simulink model "SimplificationDemo_Before"  (Simulink 7.8)
settings: Solver=ode45  StartTime=0.0  StopTime=10.0  RelTol=1e-3
settings Model: Creator=760162  LastModifiedBy=monika

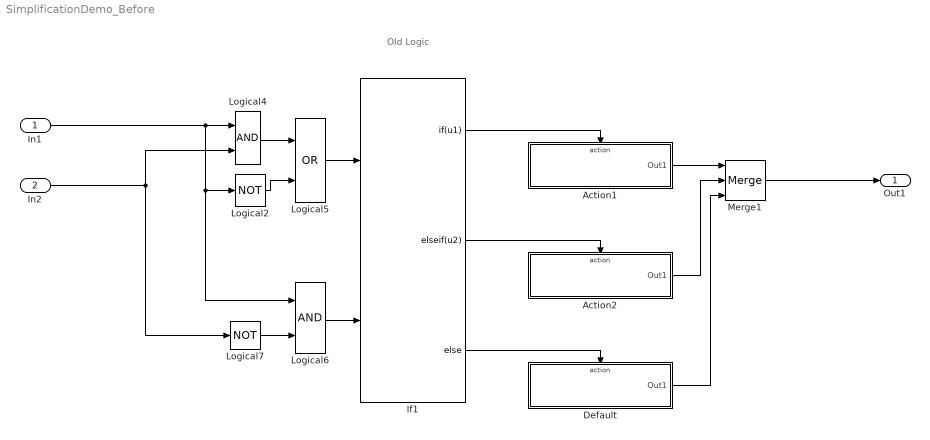
== system SimplificationDemo_Before ==
  note: Old Logic
  In1 : Inport
  In2 : Inport  Port=2
  Action1 : Subsystem  TreatAsAtomicUnit=on
      settings: CopyFcn=breaklink(gcb)  PropExecContextOutsideSubsystem=on
      mask Display:
      | text(.52,.01,char(get_param(gcb,'Tag') ), 'horizontalAlignment','center','verticalAlignment','bottom' )
      | disp(get_param(gcb,'Name'))
  Action2 : Subsystem  TreatAsAtomicUnit=on
      settings: CopyFcn=breaklink(gcb)  PropExecContextOutsideSubsystem=on
      mask Display:
      | text(.52,.01,char(get_param(gcb,'Tag') ), 'horizontalAlignment','center','verticalAlignment','bottom' )
      | disp(get_param(gcb,'Name'))
  Default : Subsystem  TreatAsAtomicUnit=on
      settings: CopyFcn=breaklink(gcb)  PropExecContextOutsideSubsystem=on
      mask Display:
      | text(.52,.01,char(get_param(gcb,'Tag') ), 'horizontalAlignment','center','verticalAlignment','bottom' )
      | disp(get_param(gcb,'Name'))
  If1 : If  NumInputs=2  IfExpression=u1  ElseIfExpressions=u2
      settings: CopyFcn=breaklink(gcb)
  Logical2 : Logic  Operator=NOT  OutDataTypeStr=boolean
  Logical4 : Logic  OutDataTypeStr=boolean
  Logical5 : Logic  Operator=OR  OutDataTypeStr=boolean
  Logical6 : Logic  OutDataTypeStr=boolean
  Logical7 : Logic  Operator=NOT  OutDataTypeStr=boolean
  Merge1 : Merge  Inputs=3
  Out1 : Outport
  wires:
  In1/1 -> Logical4/1, Logical6/1, Logical2/1
  Logical4/1 -> Logical5/1
  Logical5/1 -> If1/1
  Logical7/1 -> Logical6/2
  If1/1 -> Action1/Action
  If1/2 -> Action2/Action
  If1/3 -> Default/Action
  Logical6/1 -> If1/2
  Action1/1(Out1) -> Merge1/1
  Action2/1(Out1) -> Merge1/2
  Default/1(Out1) -> Merge1/3
  Merge1/1 -> Out1/1
  In2/1 -> Logical4/2, Logical7/1
  Logical2/1 -> Logical5/2

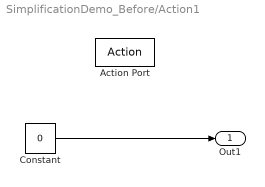
== system SimplificationDemo_Before/Action1 ==
  Action Port : ActionPort  ActionType=then
  Constant : Constant  Value=0
  Out1 : Outport
  wires:
  Constant/1 -> Out1/1

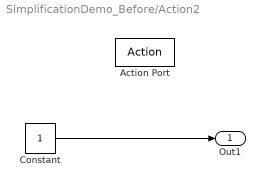
== system SimplificationDemo_Before/Action2 ==
  Action Port : ActionPort  ActionType=elseif
  Constant : Constant
  Out1 : Outport
  wires:
  Constant/1 -> Out1/1

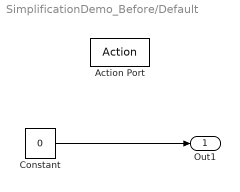
== system SimplificationDemo_Before/Default ==
  Action Port : ActionPort  ActionType=else
  Constant : Constant  Value=0
  Out1 : Outport
  wires:
  Constant/1 -> Out1/1
